simulink model "APF_CTL_VIS_Obs_2023a"  (R2023a)
settings: Solver=ode4  StartTime=0.0  StopTime=tsim  FixedStep=baseRate  RelTol=1e-6  AbsTol=1e-6
values from neighbouring files (symbols this model uses):
  A = [0 0 0 1 0 0 ... (first row only)    [CTL_NEW.m]    (also in UKF_SPOT.m = [1 0 0 dt 0 0)
  a = 25.028    [CTL_NEW.m]
  a1 = shape(1)    [Cardioid.m]    (also in Run_Initializer.m = 0.3)
  a2 = shape(2)    [Cardioid.m]    (also in Run_Initializer.m = 0.3)
  a3 = shape(3)    [Cardioid.m]    (also in Run_Initializer.m = 0.4)
  adadelta_epsilon = 1e-5    (= 1e-05)    [Run_Initializer.m]
  adadelta_gamma = 0.37    [Run_Initializer.m]
  adagrad_epsilon = 1e-8    (= 1e-08)    [Run_Initializer.m]
  adagrad_eta = 0.18    [Run_Initializer.m]
  adam_beta_1 = 0.99    [Run_Initializer.m]
  adam_beta_2 = 0.999    [Run_Initializer.m]
  adam_epsilon = 1e-2    (= 0.01)    [Run_Initializer.m]
  adam_eta = 0.0163    [Run_Initializer.m]
  adamax_beta_1 = 0.5    [Run_Initializer.m]
  adamax_beta_2 = 0.999    [Run_Initializer.m]
  adamax_eta = 0.014    [Run_Initializer.m]
  alpha_Black = 0.9    [UKF_SPOT.m]
  alpha_Blue = 0.9    [UKF_SPOT.m]
  Att_Mode = 0    [Run_Initializer.m]
  b1 = shape(4)    [Cardioid.m]    (also in Run_Initializer.m = 0.175)
  b2 = shape(5)    [Cardioid.m]    (also in Run_Initializer.m = 0.175)
  beta_Black = 2    [UKF_SPOT.m]
  beta_Blue = 20    [UKF_SPOT.m]
  Binv = inv(B)    [Run_Initializer.m]
  BLACK_end = [2, 1.4, deg2rad(368)]    [Run_Initializer.m]
  BLACK_ini = [2, 1.4, deg2rad(188), 0, 0, deg2rad(1.5)]    [Run_Initializer.m]
  BLUE_end = [1.3, 1.25, deg2rad(90)]    [Run_Initializer.m]
  BLUE_ini = [1.3, 1.25, deg2rad(270), 0, 0, deg2rad(-1.5)]    [Run_Initializer.m]
  drop_states_BLACK = BLACK_ini(1:3)    [Run_Initializer.m]
  drop_states_BLUE = BLUE_ini(1:3)    [Run_Initializer.m]
  drop_states_RED = RED_ini(1:3)    [Run_Initializer.m]
  dt = 0.01    [UKF_SPOT.m]
  end_time_black = 300    [Run_Initializer.m]
  end_time_blue = 300    [Run_Initializer.m]
  F_max = 0.22    [CTL_NEW.m]
  Gamma1_el = 0.12    [Run_Initializer.m]
  Gamma1_sh = 0.005    [Run_Initializer.m]
  Gamma1_wr = 0.025    [Run_Initializer.m]
  Gamma2_el = 5    [Run_Initializer.m]
  Gamma2_sh = 5    [Run_Initializer.m]
  Gamma2_wr = 5    [Run_Initializer.m]
  Gamma3_el = 10    [Run_Initializer.m]
  Gamma3_sh = 40    [Run_Initializer.m]
  Gamma3_wr = 40    [Run_Initializer.m]
  Gamma4_el = 0.039    [Run_Initializer.m]
  Gamma4_sh = 0.015    [Run_Initializer.m]
  Gamma4_wr = 0.029    [Run_Initializer.m]
  Gamma5_el = 800    [Run_Initializer.m]
  Gamma5_sh = 800    [Run_Initializer.m]
  Gamma5_wr = 800    [Run_Initializer.m]
  Gamma6_el = 0.000001    (= 1e-06)    [Run_Initializer.m]
  Gamma6_sh = 0.005    [Run_Initializer.m]
  Gamma6_wr = 0.02    [Run_Initializer.m]
  H = [1 0 0 0 0 0 ... (first row only)    [UKF_SPOT.m]
  home_states_BLACK = BLACK_ini(1:3)    [Run_Initializer.m]
  home_states_BLUE = BLUE_ini(1:3)    [Run_Initializer.m]
  home_states_RED = RED_ini(1:3)    [Run_Initializer.m]
  Hz = 0.01    [CTL_NEW.m]
  init_states_BLACK = BLACK_ini(1:3)    [Run_Initializer.m]
  init_states_BLUE = BLUE_ini(1:3)    [Run_Initializer.m]
  init_states_RED = RED_ini(1:3)    [Run_Initializer.m]
  J = IRED    [CTL_NEW.m]    (also in UKF_SPOT.m = 0.20184)
  k = lqr(A,B1,Q,R)    [CTL_NEW.m]
  k_1_0 = k(1,1)    [CTL_NEW.m]
  k_1_t_0 = k(3,3)    [CTL_NEW.m]
  k_2_0 = k(1,4)    [CTL_NEW.m]
  k_2_t_0 = k(3,6)    [CTL_NEW.m]
  K_a = diag([2 2 3.5])    [Run_Initializer.m]
  ka = 1    [Run_Initializer.m]
  Kd_elarm = 0.8    [Run_Initializer.m]
  Kd_sharm = 1.0    (= 1)    [Run_Initializer.m]
  Kd_t = 9.5    [CTL_NEW.m]    (also in Run_Initializer.m)
  Kd_wrarm = 0.6    [Run_Initializer.m]
  Kd_x = 28    [CTL_NEW.m]    (also in Run_Initializer.m)
  Kd_y = Kd_x    (= 28)    [CTL_NEW.m]    (also in Run_Initializer.m)
  Kp_elarm = 1.2    [Run_Initializer.m]
  Kp_sharm = 1.5    [Run_Initializer.m]
  Kp_t = 1    [CTL_NEW.m]    (also in Run_Initializer.m)
  Kp_wrarm = 2    [Run_Initializer.m]
  Kp_x = 3.5    [CTL_NEW.m]    (also in Run_Initializer.m)
  Kp_y = Kp_x    (= 3.5)    [CTL_NEW.m]    (also in Run_Initializer.m)
  kr = 2    [Run_Initializer.m]
  lambda1 = 0.4    [CTL_NEW.m]
  lambda12 = 0.4    [CTL_NEW.m]
  lambda12_t = 0.05    [CTL_NEW.m]
  lambda1_t = 0.05    [CTL_NEW.m]
  lambda2 = 0.4    [CTL_NEW.m]
  lambda2_t = 0.05    [CTL_NEW.m]
  lamda_Black = (alpha_Black^2)*(N + kappa_Black) - N    (= 15.06)    [UKF_SPOT.m]
  lamda_Blue = (alpha_Blue^2)*(N + kappa_Blue) - N    (= 6.96)    [UKF_SPOT.m]
  m = mRED    [CTL_NEW.m]    (also in UKF_SPOT.m = 11.21)
  method = 1    [UKF_SPOT.m]
  Method = 8    [Run_Initializer.m]
  momentum_eta = 0.7    [Run_Initializer.m]
  momentum_gamma = 0.7    [Run_Initializer.m]
  nesterov_eta = 0.6    [Run_Initializer.m]
  nesterov_gamma = 0.3    [Run_Initializer.m]
  Nmat = diag([1 1 1])    [Run_Initializer.m]
  p = 0.4    [CTL_NEW.m]
  P_b = diag([45 45 0])    [Run_Initializer.m]
  P_IC_Black = 0.2*eye(6)    [UKF_SPOT.m]
  P_IC_Blue = 0.2*eye(6)    [UKF_SPOT.m]
  p_t = 0.05    [CTL_NEW.m]
  psi = 1    [Run_Initializer.m]
  PWMFreq = 5    [Run_Initializer.m]
  Q = [w 0 0 0 0 0 ... (first row only)    [CTL_NEW.m]
  Q_a = diag([5, 5, 0])    [Run_Initializer.m]
  Q_b = diag([0.0125, 0.0125, 0.05])    [Run_Initializer.m]
  Q_Black = [0.0000005 0 0 0 0 0 ... (first row only)    [UKF_SPOT.m]
  Q_Blue = [0.000075 0 0 0 0 0 ... (first row only)    [UKF_SPOT.m]
  R = [r 0 0 ... (first row only)    [CTL_NEW.m]
  R_Black = [variance 0 0 ... (first row only)    [UKF_SPOT.m]
  R_Blue = [variance 0 0 ... (first row only)    [UKF_SPOT.m]
  r_hold = 0.427    [Run_Initializer.m]
  r_off = 0.165    [Run_Initializer.m]
  RED_ini = [2.7, 0.4, deg2rad(135+360), 0, 0, 0]    [Run_Initializer.m]
  Red_Rate = 0.025    [CTL_NEW.m]
  RMSprop_epsilon = 1e-8    (= 1e-08)    [Run_Initializer.m]
  RMSprop_eta = 0.025    [Run_Initializer.m]
  RMSprop_gamma = 0.9    [Run_Initializer.m]
  ... (+11 more)
undefined symbols (not defined in the file or in its folder): alpha, alpha_m, alphap, alphat, Am, b, b0, b3, baseRate, beta, Bm, c, Cm, d, DiscIntNeverNeededParam, Dm, drop_states_ARM, epsilon, F_Black_X_nominal, F_Black_Y_nominal, F_Blue_X_nominal, F_Blue_Y_nominal, F_red_X_nominal, F_red_Y_nominal, F_thrusters_BLACK, F_thrusters_BLUE, F_thrusters_RED, IBLACK, IBLUE, IDIST, IEE, IPROX, IRED, K, k1, k1t, k2, k2t, K_t, Kd_tb, Kd_tblue, Kd_tr, Kd_xb, Kd_xblue, Kd_xr, Kd_yb, Kd_yblue, Kd_yr, Kp_tb, Kp_tblue, Kp_tr, Kp_xb, Kp_xblue, Kp_xr, Kp_yb, Kp_yblue, Kp_yr, lamda ... (+34)
libraries: nvidiaSharedBlocks x10, MainLibrary x4, dspsigops x4, simulink x2, etargetslib x1
(part 4 of 15)

== system APF_CTL_VIS_Obs_2023a/Phase #2: Initial Position/Change BLACK Behavior/Custom Discrete PD (X-Position) ==
  ex : Inport
  Sum3 : Sum
  kd_xb : Gain  Gain=Kd_xb
  kp_xb : Gain  Gain=Kp_xb
  "x_dot -> x1" : Subsystem
  Fx : Outport  VectorParamsAs1DForOutWhenUnconnected=off
  wires:
  kd_xb/1 -> Sum3/1
  ex/1 -> "x_dot -> x1"/1(y(t)), kp_xb/1
  kp_xb/1 -> Sum3/2
  "x_dot -> x1"/1(dy(t)/dt) -> kd_xb/1
  Sum3/1 -> Fx/1

== system APF_CTL_VIS_Obs_2023a/Phase #2: Initial Position/Change BLACK Behavior/Custom Discrete PD (Y-Position) ==
  ey : Inport
  Sum3 : Sum
  kd_yb : Gain  Gain=Kd_yb
  kp_yb : Gain  Gain=Kp_yb
  "x_dot -> x1" : Subsystem
  Fy : Outport  VectorParamsAs1DForOutWhenUnconnected=off
  wires:
  kd_yb/1 -> Sum3/1
  Sum3/1 -> Fy/1
  kp_yb/1 -> Sum3/2
  "x_dot -> x1"/1(dy(t)/dt) -> kd_yb/1
  ey/1 -> "x_dot -> x1"/1(y(t)), kp_yb/1

== system APF_CTL_VIS_Obs_2023a/Phase #2: Initial Position/Change BLACK Behavior/Hough Control ==
  Ref : Inport
  Act : Inport  Port=2
  MATLAB Function2 : MATLAB Function  TreatAsAtomicUnit=on
  MATLAB Function3 : MATLAB Function  TreatAsAtomicUnit=on
  MATLAB Function4 : MATLAB Function  TreatAsAtomicUnit=on
  Subtract2 : Sum  Inputs=+-
  Err : Outport  VectorParamsAs1DForOutWhenUnconnected=off
  wires:
  MATLAB Function4/1(e_out) -> Err/1
  MATLAB Function2/1(Oy) -> MATLAB Function4/1(Oy)
  Subtract2/1 -> MATLAB Function4/2(e_in)
  MATLAB Function2/2(Ox) -> Subtract2/1
  Act/1 -> MATLAB Function3/1(z)
  Ref/1 -> MATLAB Function2/1(z)
  MATLAB Function3/1(Ox) -> Subtract2/2

== system APF_CTL_VIS_Obs_2023a/Phase #2: Initial Position/Change BLUE Behavior/Custom Discrete PD (Attitude) ==
  ez : Inport
  Sum3 : Sum
  kd_tb : Gain  Gain=Kd_tblue
  kp_tb : Gain  Gain=Kp_tblue
  "x_dot -> x1" : Subsystem
  Tz : Outport  VectorParamsAs1DForOutWhenUnconnected=off
  wires:
  kd_tb/1 -> Sum3/1
  Sum3/1 -> Tz/1
  kp_tb/1 -> Sum3/2
  "x_dot -> x1"/1(dy(t)/dt) -> kd_tb/1
  ez/1 -> "x_dot -> x1"/1(y(t)), kp_tb/1

== system APF_CTL_VIS_Obs_2023a/Phase #2: Initial Position/Change BLUE Behavior/Custom Discrete PD (X-Position) ==
  ex : Inport
  Sum3 : Sum
  kd_xb : Gain  Gain=Kd_xblue
  kp_xb : Gain  Gain=Kp_xblue
  "x_dot -> x1" : Subsystem
  Fx : Outport  VectorParamsAs1DForOutWhenUnconnected=off
  wires:
  kd_xb/1 -> Sum3/1
  ex/1 -> "x_dot -> x1"/1(y(t)), kp_xb/1
  kp_xb/1 -> Sum3/2
  "x_dot -> x1"/1(dy(t)/dt) -> kd_xb/1
  Sum3/1 -> Fx/1

== system APF_CTL_VIS_Obs_2023a/Phase #2: Initial Position/Change BLUE Behavior/Custom Discrete PD (Y-Position) ==
  ey : Inport
  Sum3 : Sum
  kd_yb : Gain  Gain=Kd_yblue
  kp_yb : Gain  Gain=Kp_yblue
  "x_dot -> x1" : Subsystem
  Fy : Outport  VectorParamsAs1DForOutWhenUnconnected=off
  wires:
  kd_yb/1 -> Sum3/1
  Sum3/1 -> Fy/1
  kp_yb/1 -> Sum3/2
  "x_dot -> x1"/1(dy(t)/dt) -> kd_yb/1
  ey/1 -> "x_dot -> x1"/1(y(t)), kp_yb/1

== system APF_CTL_VIS_Obs_2023a/Phase #2: Initial Position/Change BLUE Behavior/Hough Control ==
  Ref : Inport
  Act : Inport  Port=2
  MATLAB Function2 : MATLAB Function  TreatAsAtomicUnit=on
  MATLAB Function3 : MATLAB Function  TreatAsAtomicUnit=on
  MATLAB Function4 : MATLAB Function  TreatAsAtomicUnit=on
  Subtract2 : Sum  Inputs=+-
  Err : Outport  VectorParamsAs1DForOutWhenUnconnected=off
  wires:
  MATLAB Function4/1(e_out) -> Err/1
  MATLAB Function2/1(Oy) -> MATLAB Function4/1(Oy)
  Subtract2/1 -> MATLAB Function4/2(e_in)
  MATLAB Function2/2(Ox) -> Subtract2/1
  Act/1 -> MATLAB Function3/1(z)
  Ref/1 -> MATLAB Function2/1(z)
  MATLAB Function3/1(Ox) -> Subtract2/2

== system APF_CTL_VIS_Obs_2023a/Phase #2: Initial Position/Change RED Behavior/Custom Discrete PD (Attitude) ==
  ez : Inport
  Sum3 : Sum
  kd_tr : Gain  Gain=Kd_tr
  kp_tr : Gain  Gain=Kp_tr
  "x_dot -> x2" : Subsystem
  Tz : Outport  VectorParamsAs1DForOutWhenUnconnected=off
  wires:
  kd_tr/1 -> Sum3/1
  Sum3/1 -> Tz/1
  kp_tr/1 -> Sum3/2
  "x_dot -> x2"/1(dy(t)/dt) -> kd_tr/1
  ez/1 -> "x_dot -> x2"/1(y(t)), kp_tr/1

== system APF_CTL_VIS_Obs_2023a/Phase #2: Initial Position/Change RED Behavior/Custom Discrete PD (X-Position) ==
  ex : Inport
  Sum3 : Sum
  kd_xr : Gain  Gain=Kd_xr
  kp_xr : Gain  Gain=Kp_xr
  "x_dot -> x2" : Subsystem
  Fx : Outport  VectorParamsAs1DForOutWhenUnconnected=off
  wires:
  kd_xr/1 -> Sum3/1
  ex/1 -> "x_dot -> x2"/1(y(t)), kp_xr/1
  kp_xr/1 -> Sum3/2
  "x_dot -> x2"/1(dy(t)/dt) -> kd_xr/1
  Sum3/1 -> Fx/1

== system APF_CTL_VIS_Obs_2023a/Phase #2: Initial Position/Change RED Behavior/Custom Discrete PD (Y-Position) ==
  ey : Inport
  Sum3 : Sum
  kd_yr : Gain  Gain=Kd_yr
  kp_yr : Gain  Gain=Kp_yr
  "x_dot -> x2" : Subsystem
  Fy : Outport  VectorParamsAs1DForOutWhenUnconnected=off
  wires:
  kd_yr/1 -> Sum3/1
  Sum3/1 -> Fy/1
  kp_yr/1 -> Sum3/2
  "x_dot -> x2"/1(dy(t)/dt) -> kd_yr/1
  ey/1 -> "x_dot -> x2"/1(y(t)), kp_yr/1

== system APF_CTL_VIS_Obs_2023a/Phase #2: Initial Position/Change RED Behavior/Hough Control ==
  Ref : Inport
  Act : Inport  Port=2
  MATLAB Function2 : MATLAB Function  TreatAsAtomicUnit=on
  MATLAB Function3 : MATLAB Function  TreatAsAtomicUnit=on
  MATLAB Function4 : MATLAB Function  TreatAsAtomicUnit=on
  Subtract2 : Sum  Inputs=+-
  Err : Outport  VectorParamsAs1DForOutWhenUnconnected=off
  wires:
  MATLAB Function4/1(e_out) -> Err/1
  MATLAB Function2/1(Oy) -> MATLAB Function4/1(Oy)
  Subtract2/1 -> MATLAB Function4/2(e_in)
  MATLAB Function2/2(Ox) -> Subtract2/1
  Act/1 -> MATLAB Function3/1(z)
  Ref/1 -> MATLAB Function2/1(z)
  MATLAB Function3/1(Ox) -> Subtract2/2

== system APF_CTL_VIS_Obs_2023a/Phase #2: Initial Position/Change RED Behavior/RED+ARM ==
  note: ARM Control Law - RED
  note: This section is reserved for any control law for the robotic manipulator.
  Action Port : ActionPort  ActionPortLabel=if(u1 == 4 | u1 == 5 | u1 == 10 | u1 == 11)
  Constant4 : Constant  Value=pi/2
  Constant5 : Constant  Value=pi/2
  Constant6 : Constant  Value=0
  Constant7 : Constant
  Data Store Read1 : DataStoreRead  DataStoreName=isSim  IndexOptions=Index vector (dialog)  Indices=1  OutputSizes=1
  Data Store Write : DataStoreWrite  DataStoreName=RED_Shoulder_Command  IndexOptions=Index vector (dialog)  Indices=1  OutputSizes=1
  Data Store Write1 : DataStoreWrite  DataStoreName=RED_Elbow_Command  IndexOptions=Index vector (dialog)  Indices=1  OutputSizes=1
  Data Store Write2 : DataStoreWrite  DataStoreName=RED_Wrist_Command  IndexOptions=Index vector (dialog)  Indices=1  OutputSizes=1
  Data Store Write3 : DataStoreWrite  DataStoreName=RED_ARM_Control_Mode  IndexOptions=Index vector (dialog)  Indices=1  OutputSizes=1
  "If 'simMode' set to '1', then this is a simulation and the dynamics will be simulated. Otherwise, this is an experiment, and the simulation will not be run." : If  IfExpression=u1 == 1
  Merge : Merge
  Merge1 : Merge
  Merge2 : Merge
  Passthrough for Experiment : Subsystem  TreatAsAtomicUnit=on
  Simulated Position Controller : Subsystem  TreatAsAtomicUnit=on
  wires:
  Constant7/1 -> Data Store Write3/1
  Constant6/1 -> Passthrough for Experiment/3(q3_desired), Simulated Position Controller/3(q3_desired)
  Constant4/1 -> Passthrough for Experiment/1(q1_desired), Simulated Position Controller/1(q1_desired)
  Constant5/1 -> Passthrough for Experiment/2(q2_desired), Simulated Position Controller/2(q2_desired)
  Data Store Read1/1 -> "If 'simMode' set to '1', then this is a simulation and the dynamics will be simulated. Otherwise, this is an experiment, and the simulation will not be run."/1
  "If 'simMode' set to '1', then this is a simulation and the dynamics will be simulated. Otherwise, this is an experiment, and the simulation will not be run."/1 -> Simulated Position Controller/Action
  "If 'simMode' set to '1', then this is a simulation and the dynamics will be simulated. Otherwise, this is an experiment, and the simulation will not be run."/2 -> Passthrough for Experiment/Action
  Simulated Position Controller/1(q1_command) -> Merge/1
  Passthrough for Experiment/1(q1_command) -> Merge/2
  Merge/1 -> Data Store Write/1
  Simulated Position Controller/2(q2_command) -> Merge1/1
  Merge1/1 -> Data Store Write1/1
  Passthrough for Experiment/2(q2_command) -> Merge1/2
  Simulated Position Controller/3(q3_command) -> Merge2/1
  Passthrough for Experiment/3(q3_command) -> Merge2/2
  Merge2/1 -> Data Store Write2/1

== system APF_CTL_VIS_Obs_2023a/Phase #3: Experiment/Change BLACK Behavior/Sub-Phase #1 ==
  note: PD Control Law - BLACK
  note: Additional Blocks
  note: A simple PD control law is used here to command the platform to it's initial position, as defined in the initializer.
  note: Additional blocks are stored here.
  Action Port : ActionPort  ActionPortLabel=if(u1 < u2)
  BLACK_Fx : DataStoreWrite  DataStoreName=BLACK_Fx  IndexOptions=Index vector (dialog)  Indices=1  OutputSizes=1
  BLACK_Fy : DataStoreWrite  DataStoreName=BLACK_Fy  IndexOptions=Index vector (dialog)  Indices=1  OutputSizes=1
  BLACK_Px : DataStoreRead  DataStoreName=BLACK_Px  IndexOptions=Index vector (dialog)  Indices=1  OutputSizes=1
  "BLACK_Py " : DataStoreRead  DataStoreName=BLACK_Py  IndexOptions=Index vector (dialog)  Indices=1  OutputSizes=1
  BLACK_Rz : DataStoreRead  DataStoreName=BLACK_Rz  IndexOptions=Index vector (dialog)  Indices=1  OutputSizes=1
  BLACK_Rz Desired : Subsystem
  BLACK_Tz : DataStoreWrite  DataStoreName=BLACK_Tz  IndexOptions=Index vector (dialog)  Indices=1  OutputSizes=1
  Custom Discrete PD (Attitude) : Subsystem
  Custom Discrete PD (X-Position) : Subsystem
  Custom Discrete PD (Y-Position) : Subsystem
  Data Store Write3 : DataStoreWrite  DataStoreName=Float_State  IndexOptions=Index vector (dialog)  Indices=1  OutputSizes=1
  Desired X-Position (BLACK) : Constant  Value=xLength/2  SampleTime=-1
  Desired Y-Position (BLACK) : Constant  Value=yLength/2  SampleTime=-1
  Hough Control : Subsystem
  Puck State : Constant
  Subtract : Sum  Inputs=+-
  Subtract1 : Sum  Inputs=+-
  wires:
  Puck State/1 -> Data Store Write3/1
  "BLACK_Py "/1 -> Subtract1/2
  Desired X-Position (BLACK)/1 -> Subtract/1
  BLACK_Rz Desired/1(Out1) -> Hough Control/1(Ref)
  Custom Discrete PD (X-Position)/1(Fx) -> BLACK_Fx/1
  Desired Y-Position (BLACK)/1 -> Subtract1/1
  Hough Control/1(Err) -> Custom Discrete PD (Attitude)/1(ez)
  Subtract/1 -> Custom Discrete PD (X-Position)/1(ex)
  Custom Discrete PD (Y-Position)/1(Fy) -> BLACK_Fy/1
  Subtract1/1 -> Custom Discrete PD (Y-Position)/1(ey)
  Custom Discrete PD (Attitude)/1(Tz) -> BLACK_Tz/1
  BLACK_Rz/1 -> Hough Control/2(Act)
  BLACK_Px/1 -> Subtract/2

== system APF_CTL_VIS_Obs_2023a/Phase #3: Experiment/Change BLACK Behavior/Sub-Phase #2  ==
  note: PD Control Law - BLACK
  note: Additional Blocks
  note: Additional blocks are stored here.
  Action Port : ActionPort  ActionPortLabel=elseif((u1 < u3 & u1 >= u2))
  BLACK_Fx : DataStoreWrite  DataStoreName=BLACK_Fx  IndexOptions=Index vector (dialog)  Indices=1  OutputSizes=1
  BLACK_Fy : DataStoreWrite  DataStoreName=BLACK_Fy  IndexOptions=Index vector (dialog)  Indices=1  OutputSizes=1
  BLACK_Px : DataStoreRead  DataStoreName=BLACK_Px  IndexOptions=Index vector (dialog)  Indices=1  OutputSizes=1
  "BLACK_Py " : DataStoreRead  DataStoreName=BLACK_Py  IndexOptions=Index vector (dialog)  Indices=1  OutputSizes=1
  BLACK_Rz : DataStoreRead  DataStoreName=BLACK_Rz  IndexOptions=Index vector (dialog)  Indices=1  OutputSizes=1
  BLACK_Rz Desired : Subsystem
  BLACK_Tz : DataStoreWrite  DataStoreName=BLACK_Tz  IndexOptions=Index vector (dialog)  Indices=1  OutputSizes=1
  Custom Discrete PD (Attitude) : Subsystem
  Custom Discrete PD (X-Position) : Subsystem
  Custom Discrete PD (Y-Position) : Subsystem
  Data Store Write3 : DataStoreWrite  DataStoreName=Float_State  IndexOptions=Index vector (dialog)  Indices=1  OutputSizes=1
  Desired X-Position (BLACK) : Constant  Value=xLength/2  SampleTime=-1
  Desired Y-Position (BLACK) : Constant  Value=yLength/2  SampleTime=-1
  Hough Control : Subsystem
  Puck State : Constant
  Subtract : Sum  Inputs=+-
  Subtract1 : Sum  Inputs=+-
  wires:
  Puck State/1 -> Data Store Write3/1
  BLACK_Px/1 -> Subtract/2
  Custom Discrete PD (Y-Position)/1(Fy) -> BLACK_Fy/1
  Subtract/1 -> Custom Discrete PD (X-Position)/1(ex)
  Desired Y-Position (BLACK)/1 -> Subtract1/1
  Custom Discrete PD (Attitude)/1(Tz) -> BLACK_Tz/1
  Subtract1/1 -> Custom Discrete PD (Y-Position)/1(ey)
  BLACK_Rz/1 -> Hough Control/2(Act)
  Custom Discrete PD (X-Position)/1(Fx) -> BLACK_Fx/1
  Hough Control/1(Err) -> Custom Discrete PD (Attitude)/1(ez)
  "BLACK_Py "/1 -> Subtract1/2
  Desired X-Position (BLACK)/1 -> Subtract/1
  BLACK_Rz Desired/1(Out1) -> Hough Control/1(Ref)

== system APF_CTL_VIS_Obs_2023a/Phase #3: Experiment/Change BLACK Behavior/Sub-Phase #3  ==
  note: PD Control Law - BLACK
  note: Additional Blocks
  note: Additional blocks are stored here.
  Action Port : ActionPort  ActionPortLabel=elseif((u1 < u4 & u1 >= u3))
  BLACK_Fx : DataStoreWrite  DataStoreName=BLACK_Fx  IndexOptions=Index vector (dialog)  Indices=1  OutputSizes=1
  BLACK_Fy : DataStoreWrite  DataStoreName=BLACK_Fy  IndexOptions=Index vector (dialog)  Indices=1  OutputSizes=1
  BLACK_Px : DataStoreRead  DataStoreName=BLACK_Px  IndexOptions=Index vector (dialog)  Indices=1  OutputSizes=1
  "BLACK_Py " : DataStoreRead  DataStoreName=BLACK_Py  IndexOptions=Index vector (dialog)  Indices=1  OutputSizes=1
  BLACK_Rz : DataStoreRead  DataStoreName=BLACK_Rz  IndexOptions=Index vector (dialog)  Indices=1  OutputSizes=1
  BLACK_Rz Desired : Subsystem
  BLACK_Tz : DataStoreWrite  DataStoreName=BLACK_Tz  IndexOptions=Index vector (dialog)  Indices=1  OutputSizes=1
  Custom Discrete PD (Attitude) : Subsystem
  Custom Discrete PD (X-Position) : Subsystem
  Custom Discrete PD (Y-Position) : Subsystem
  Data Store Write3 : DataStoreWrite  DataStoreName=Float_State  IndexOptions=Index vector (dialog)  Indices=1  OutputSizes=1
  Desired X-Position (BLACK) : Constant  Value=xLength/2  SampleTime=-1
  Desired Y-Position (BLACK) : Constant  Value=yLength/2  SampleTime=-1
  Hough Control : Subsystem
  Puck State : Constant
  Subtract : Sum  Inputs=+-
  Subtract1 : Sum  Inputs=+-
  wires:
  Puck State/1 -> Data Store Write3/1
  BLACK_Px/1 -> Subtract/2
  Custom Discrete PD (Y-Position)/1(Fy) -> BLACK_Fy/1
  Subtract/1 -> Custom Discrete PD (X-Position)/1(ex)
  Desired Y-Position (BLACK)/1 -> Subtract1/1
  Custom Discrete PD (Attitude)/1(Tz) -> BLACK_Tz/1
  Subtract1/1 -> Custom Discrete PD (Y-Position)/1(ey)
  BLACK_Rz/1 -> Hough Control/2(Act)
  Custom Discrete PD (X-Position)/1(Fx) -> BLACK_Fx/1
  Hough Control/1(Err) -> Custom Discrete PD (Attitude)/1(ez)
  "BLACK_Py "/1 -> Subtract1/2
  Desired X-Position (BLACK)/1 -> Subtract/1
  BLACK_Rz Desired/1(Out1) -> Hough Control/1(Ref)

== system APF_CTL_VIS_Obs_2023a/Phase #3: Experiment/Change BLACK Behavior/Sub-Phase #4 ==
  note: PD Control Law - BLACK
  note: Additional Blocks
  note: A simple PD control law is used here to command the platform to it's initial position, as defined in the initializer.
  note: Additional blocks are stored here.
  Action Port : ActionPort  ActionPortLabel=elseif( (u1 < u5 & u1 >= u4))
  BLACK_Fx : DataStoreWrite  DataStoreName=BLACK_Fx  IndexOptions=Index vector (dialog)  Indices=1  OutputSizes=1
  BLACK_Fy : DataStoreWrite  DataStoreName=BLACK_Fy  IndexOptions=Index vector (dialog)  Indices=1  OutputSizes=1
  BLACK_Px : DataStoreRead  DataStoreName=BLACK_Px  IndexOptions=Index vector (dialog)  Indices=1  OutputSizes=1
  "BLACK_Py " : DataStoreRead  DataStoreName=BLACK_Py  IndexOptions=Index vector (dialog)  Indices=1  OutputSizes=1
  BLACK_Rz : DataStoreRead  DataStoreName=BLACK_Rz  IndexOptions=Index vector (dialog)  Indices=1  OutputSizes=1
  BLACK_RzD : Subsystem  Commented=on
  BLACK_Tz : DataStoreWrite  DataStoreName=BLACK_Tz  IndexOptions=Index vector (dialog)  Indices=1  OutputSizes=1
  Custom Discrete PD (Attitude) : Subsystem
  Custom Discrete PD (X-Position) : Subsystem
  Custom Discrete PD (Y-Position) : Subsystem
  Data Store Write3 : DataStoreWrite  DataStoreName=Float_State  IndexOptions=Index vector (dialog)  Indices=1  OutputSizes=1
  Hough Control : Subsystem
  Motion X1 : Subsystem
  Motion Y1 : Subsystem
  Motion Z1 : Subsystem
  Puck State : Constant
  Subtract : Sum  Inputs=+-
  Subtract1 : Sum  Inputs=+-
  wires:
  Puck State/1 -> Data Store Write3/1
  BLACK_Rz/1 -> Hough Control/2(Act)
  Subtract1/1 -> Custom Discrete PD (Y-Position)/1(ey)
  Hough Control/1(Err) -> Custom Discrete PD (Attitude)/1(ez)
  "BLACK_Py "/1 -> Subtract1/2
  BLACK_Px/1 -> Subtract/2
  Subtract/1 -> Custom Discrete PD (X-Position)/1(ex)
  Custom Discrete PD (Attitude)/1(Tz) -> BLACK_Tz/1
  Custom Discrete PD (Y-Position)/1(Fy) -> BLACK_Fy/1
  Custom Discrete PD (X-Position)/1(Fx) -> BLACK_Fx/1
  Motion X1/1(Out1) -> Subtract/1
  Motion Y1/1(Out1) -> Subtract1/1
  Motion Z1/1(Ref) -> Hough Control/1(Ref)

== system APF_CTL_VIS_Obs_2023a/Phase #3: Experiment/Change BLUE Behavior/Sub-Phase #1 ==
  note: PD Control Law - BLUE
  note: A simple PD control law is used here to command the platform to it's initial position, as defined in the initializer.
  note: Additional Blocks
  note: Additional blocks are stored here.
  Action Port : ActionPort  ActionPortLabel=if(u1 < u2)
  BLUE_Fx : DataStoreWrite  DataStoreName=BLUE_Fx  IndexOptions=Index vector (dialog)  Indices=1  OutputSizes=1
  BLUE_Fy : DataStoreWrite  DataStoreName=BLUE_Fy  IndexOptions=Index vector (dialog)  Indices=1  OutputSizes=1
  BLUE_Px : DataStoreRead  DataStoreName=BLUE_Px  IndexOptions=Index vector (dialog)  Indices=1  OutputSizes=1
  "BLUE_Py " : DataStoreRead  DataStoreName=BLUE_Py  IndexOptions=Index vector (dialog)  Indices=1  OutputSizes=1
  BLUE_Rz : DataStoreRead  DataStoreName=BLUE_Rz  IndexOptions=Index vector (dialog)  Indices=1  OutputSizes=1
  BLUE_Rz Desired : Subsystem
  BLUE_Tz : DataStoreWrite  DataStoreName=BLUE_Tz  IndexOptions=Index vector (dialog)  Indices=1  OutputSizes=1
  Custom Discrete PD (Attitude) : Subsystem
  Custom Discrete PD (X-Position) : Subsystem
  Custom Discrete PD (Y-Position) : Subsystem
  Data Store Write1 : DataStoreWrite  DataStoreName=Float_State  IndexOptions=Index vector (dialog)  Indices=1  OutputSizes=1
  Hough Control : Subsystem
  MATLAB Function2 : MATLAB Function  TreatAsAtomicUnit=on
  MATLAB Function3 : MATLAB Function  TreatAsAtomicUnit=on
  Puck State : Constant
  Subsystem2 : Subsystem
  Subtract : Sum  Inputs=+-
  Subtract1 : Sum  Inputs=+-
  wires:
  Puck State/1 -> Data Store Write1/1
  Custom Discrete PD (Attitude)/1(Tz) -> BLUE_Tz/1
  MATLAB Function3/1(y) -> Subtract1/1
  MATLAB Function2/1(x) -> Subtract/1
  Hough Control/1(Err) -> Custom Discrete PD (Attitude)/1(ez)
  BLUE_Rz/1 -> Hough Control/2(Act)
  Custom Discrete PD (Y-Position)/1(Fy) -> BLUE_Fy/1
  Subtract/1 -> Custom Discrete PD (X-Position)/1(ex)
  BLUE_Px/1 -> Subtract/2
  Custom Discrete PD (X-Position)/1(Fx) -> BLUE_Fx/1
  Subsystem2/1(Out1) -> MATLAB Function2/1(t), MATLAB Function3/1(t)
  Subtract1/1 -> Custom Discrete PD (Y-Position)/1(ey)
  "BLUE_Py "/1 -> Subtract1/2
  BLUE_Rz Desired/1(Ref) -> Hough Control/1(Ref)

== system APF_CTL_VIS_Obs_2023a/Phase #3: Experiment/Change BLUE Behavior/Sub-Phase #2  ==
  note: Additional blocks are stored here.
  note: A simple PD control law is used here to command the platform to it's initial position, as defined in the initializer.
  note: Additional Blocks
  note: PD Control Law - BLUE
  Action Port : ActionPort  ActionPortLabel=elseif((u1 < u3 & u1 >= u2))
  BLUE_Fx : DataStoreWrite  DataStoreName=BLUE_Fx  IndexOptions=Index vector (dialog)  Indices=1  OutputSizes=1
  BLUE_Fy : DataStoreWrite  DataStoreName=BLUE_Fy  IndexOptions=Index vector (dialog)  Indices=1  OutputSizes=1
  BLUE_Px : DataStoreRead  DataStoreName=BLUE_Px  IndexOptions=Index vector (dialog)  Indices=1  OutputSizes=1
  "BLUE_Py " : DataStoreRead  DataStoreName=BLUE_Py  IndexOptions=Index vector (dialog)  Indices=1  OutputSizes=1
  BLUE_Rz : DataStoreRead  DataStoreName=BLUE_Rz  IndexOptions=Index vector (dialog)  Indices=1  OutputSizes=1
  BLUE_Rz Desired : Subsystem
  BLUE_Tz : DataStoreWrite  DataStoreName=BLUE_Tz  IndexOptions=Index vector (dialog)  Indices=1  OutputSizes=1
  Custom Discrete PD (Attitude) : Subsystem
  Custom Discrete PD (X-Position) : Subsystem
  Custom Discrete PD (Y-Position) : Subsystem
  Data Store Write1 : DataStoreWrite  DataStoreName=Float_State  IndexOptions=Index vector (dialog)  Indices=1  OutputSizes=1
  Hough Control : Subsystem
  MATLAB Function2 : MATLAB Function  TreatAsAtomicUnit=on
  MATLAB Function3 : MATLAB Function  TreatAsAtomicUnit=on
  Puck State : Constant
  Subsystem2 : Subsystem
  Subtract : Sum  Inputs=+-
  Subtract1 : Sum  Inputs=+-
  wires:
  Puck State/1 -> Data Store Write1/1
  BLUE_Rz/1 -> Hough Control/2(Act)
  BLUE_Rz Desired/1(Ref) -> Hough Control/1(Ref)
  Custom Discrete PD (Y-Position)/1(Fy) -> BLUE_Fy/1
  Subtract/1 -> Custom Discrete PD (X-Position)/1(ex)
  Subtract1/1 -> Custom Discrete PD (Y-Position)/1(ey)
  BLUE_Px/1 -> Subtract/2
  Custom Discrete PD (X-Position)/1(Fx) -> BLUE_Fx/1
  "BLUE_Py "/1 -> Subtract1/2
  Subsystem2/1(Out1) -> MATLAB Function2/1(t), MATLAB Function3/1(t)
  MATLAB Function2/1(x) -> Subtract/1
  Hough Control/1(Err) -> Custom Discrete PD (Attitude)/1(ez)
  MATLAB Function3/1(y) -> Subtract1/1
  Custom Discrete PD (Attitude)/1(Tz) -> BLUE_Tz/1

== system APF_CTL_VIS_Obs_2023a/Phase #3: Experiment/Change BLUE Behavior/Sub-Phase #3  ==
  note: Additional blocks are stored here.
  note: A simple PD control law is used here to command the platform to it's initial position, as defined in the initializer.
  note: Additional Blocks
  note: PD Control Law - BLUE
  Action Port : ActionPort  ActionPortLabel=elseif((u1 < u4 & u1 >= u3))
  BLUE_Fx : DataStoreWrite  DataStoreName=BLUE_Fx  IndexOptions=Index vector (dialog)  Indices=1  OutputSizes=1
  BLUE_Fy : DataStoreWrite  DataStoreName=BLUE_Fy  IndexOptions=Index vector (dialog)  Indices=1  OutputSizes=1
  BLUE_Px : DataStoreRead  DataStoreName=BLUE_Px  IndexOptions=Index vector (dialog)  Indices=1  OutputSizes=1
  "BLUE_Py " : DataStoreRead  DataStoreName=BLUE_Py  IndexOptions=Index vector (dialog)  Indices=1  OutputSizes=1
  BLUE_Rz : DataStoreRead  DataStoreName=BLUE_Rz  IndexOptions=Index vector (dialog)  Indices=1  OutputSizes=1
  BLUE_Rz Desired : Subsystem
  BLUE_Tz : DataStoreWrite  DataStoreName=BLUE_Tz  IndexOptions=Index vector (dialog)  Indices=1  OutputSizes=1
  Custom Discrete PD (Attitude) : Subsystem
  Custom Discrete PD (X-Position) : Subsystem
  Custom Discrete PD (Y-Position) : Subsystem
  Data Store Write1 : DataStoreWrite  DataStoreName=Float_State  IndexOptions=Index vector (dialog)  Indices=1  OutputSizes=1
  Hough Control : Subsystem
  MATLAB Function2 : MATLAB Function  TreatAsAtomicUnit=on
  MATLAB Function3 : MATLAB Function  TreatAsAtomicUnit=on
  Puck State : Constant
  Subsystem2 : Subsystem
  Subtract : Sum  Inputs=+-
  Subtract1 : Sum  Inputs=+-
  wires:
  Puck State/1 -> Data Store Write1/1
  BLUE_Rz/1 -> Hough Control/2(Act)
  BLUE_Rz Desired/1(Ref) -> Hough Control/1(Ref)
  Custom Discrete PD (Y-Position)/1(Fy) -> BLUE_Fy/1
  Subtract/1 -> Custom Discrete PD (X-Position)/1(ex)
  Subtract1/1 -> Custom Discrete PD (Y-Position)/1(ey)
  BLUE_Px/1 -> Subtract/2
  Custom Discrete PD (X-Position)/1(Fx) -> BLUE_Fx/1
  "BLUE_Py "/1 -> Subtract1/2
  Subsystem2/1(Out1) -> MATLAB Function2/1(t), MATLAB Function3/1(t)
  MATLAB Function2/1(x) -> Subtract/1
  Hough Control/1(Err) -> Custom Discrete PD (Attitude)/1(ez)
  MATLAB Function3/1(y) -> Subtract1/1
  Custom Discrete PD (Attitude)/1(Tz) -> BLUE_Tz/1

== system APF_CTL_VIS_Obs_2023a/Phase #3: Experiment/Change BLUE Behavior/Sub-Phase #4 ==
  note: Additional blocks are stored here.
  note: A simple PD control law is used here to command the platform to it's initial position, as defined in the initializer.
  note: Additional Blocks
  note: PD Control Law - BLUE
  Action Port : ActionPort  ActionPortLabel=elseif( (u1 < u5 & u1 >= u4))
  BLUE_Fx : DataStoreWrite  DataStoreName=BLUE_Fx  IndexOptions=Index vector (dialog)  Indices=1  OutputSizes=1
  BLUE_Fy : DataStoreWrite  DataStoreName=BLUE_Fy  IndexOptions=Index vector (dialog)  Indices=1  OutputSizes=1
  BLUE_Px : DataStoreRead  DataStoreName=BLUE_Px  IndexOptions=Index vector (dialog)  Indices=1  OutputSizes=1
  "BLUE_Py " : DataStoreRead  DataStoreName=BLUE_Py  IndexOptions=Index vector (dialog)  Indices=1  OutputSizes=1
  BLUE_Rz : DataStoreRead  Commented=on  DataStoreName=BLUE_Rz  IndexOptions=Index vector (dialog)  Indices=1  OutputSizes=1
  BLUE_Rz Desired : Subsystem  Commented=on
  BLUE_Tz : DataStoreWrite  DataStoreName=BLUE_Tz  IndexOptions=Index vector (dialog)  Indices=1  OutputSizes=1
  Custom Discrete PD (Attitude) : Subsystem
  Custom Discrete PD (X-Position) : Subsystem
  Custom Discrete PD (Y-Position) : Subsystem
  Data Store Read : DataStoreRead  DataStoreName=BLUE_Rz  IndexOptions=Index vector (dialog)  Indices=1  OutputSizes=1
  Data Store Write1 : DataStoreWrite  DataStoreName=Float_State  IndexOptions=Index vector (dialog)  Indices=1  OutputSizes=1
  Hough Control : Subsystem
  Motion X : Subsystem
  Motion Y : Subsystem
  Motion Z : Subsystem
  Puck State : Constant
  Subtract : Sum  Inputs=+-
  Subtract1 : Sum  Inputs=+-
  wires:
  Puck State/1 -> Data Store Write1/1
  Data Store Read/1 -> Hough Control/2(Act)
  Custom Discrete PD (Attitude)/1(Tz) -> BLUE_Tz/1
  Subtract1/1 -> Custom Discrete PD (Y-Position)/1(ey)
  Hough Control/1(Err) -> Custom Discrete PD (Attitude)/1(ez)
  Custom Discrete PD (X-Position)/1(Fx) -> BLUE_Fx/1
  BLUE_Px/1 -> Subtract/2
  Subtract/1 -> Custom Discrete PD (X-Position)/1(ex)
  Custom Discrete PD (Y-Position)/1(Fy) -> BLUE_Fy/1
  "BLUE_Py "/1 -> Subtract1/2
  Motion X/1(Out1) -> Subtract/1
  Motion Y/1(Out1) -> Subtract1/1
  Motion Z/1(Ref) -> Hough Control/1(Ref)

== system APF_CTL_VIS_Obs_2023a/Phase #3: Experiment/Change RED Behavior/Sub-Phase #1 ==
  note: PD Control Law - RED
  note: Additional Blocks
  note: Additional blocks are stored above. Note that to control attitude using the RW, simply replace RED_Tz with RED_Tz_RW.
  note: A simple PD control law is used here to command the platform to it's initial position, as defined in the initializer.
  note: ARM Control Law - RED
  Action Port : ActionPort  ActionPortLabel=if(u1 < u2)
  Constant1 : Constant  Value=0
  Constant4 : Constant  Value=platformSelection
  Custom Discrete PD (Attitude) : Subsystem
  Custom Discrete PD (X-Position) : Subsystem
  Custom Discrete PD (Y-Position) : Subsystem
  Data Store Write3 : DataStoreWrite  DataStoreName=Float_State  IndexOptions=Index vector (dialog)  Indices=1  OutputSizes=1
  Hough Control : Subsystem
  If : If  IfExpression=u1 == 4 | u1 == 5 | u1 == 10 | u1 == 11  ShowElse=off
  MATLAB Function : MATLAB Function  TreatAsAtomicUnit=on
  MATLAB Function1 : MATLAB Function  TreatAsAtomicUnit=on
  Puck State : Constant
  RED+ARM : Subsystem  TreatAsAtomicUnit=on
  RED_Fx : DataStoreWrite  DataStoreName=RED_Fx  IndexOptions=Index vector (dialog)  Indices=1  OutputSizes=1
  RED_Fy : DataStoreWrite  DataStoreName=RED_Fy  IndexOptions=Index vector (dialog)  Indices=1  OutputSizes=1
  RED_Px1 : DataStoreRead  DataStoreName=RED_Px  IndexOptions=Index vector (dialog)  Indices=1  OutputSizes=1
  "RED_Py " : DataStoreRead  DataStoreName=RED_Py  IndexOptions=Index vector (dialog)  Indices=1  OutputSizes=1
  RED_Rz : DataStoreRead  DataStoreName=RED_Rz  IndexOptions=Index vector (dialog)  Indices=1  OutputSizes=1
  RED_Rz Desired : Subsystem
  RED_Tz : DataStoreWrite  DataStoreName=RED_Tz  IndexOptions=Index vector (dialog)  Indices=1  OutputSizes=1
  RED_Tz_RW : DataStoreWrite  DataStoreName=RED_Tz_RW  IndexOptions=Index vector (dialog)  Indices=1  OutputSizes=1
  Subsystem1 : Subsystem
  Subtract : Sum  Inputs=+-
  Subtract2 : Sum  Inputs=+-
  wires:
  Constant1/1 -> RED_Tz_RW/1
  Puck State/1 -> Data Store Write3/1
  If/1 -> RED+ARM/Action
  Constant4/1 -> If/1
  Subsystem1/1(Out1) -> MATLAB Function/1(t), MATLAB Function1/1(t)
  Hough Control/1(Err) -> Custom Discrete PD (Attitude)/1(ez)
  "RED_Py "/1 -> Subtract2/2
  Custom Discrete PD (Y-Position)/1(Fy) -> RED_Fy/1
  Custom Discrete PD (Attitude)/1(Tz) -> RED_Tz/1
  RED_Px1/1 -> Subtract/2
  MATLAB Function/1(x) -> Subtract/1
  RED_Rz Desired/1(Ref) -> Hough Control/1(Ref)
  Custom Discrete PD (X-Position)/1(Fx) -> RED_Fx/1
  Subtract/1 -> Custom Discrete PD (X-Position)/1(ex)
  MATLAB Function1/1(y) -> Subtract2/1
  Subtract2/1 -> Custom Discrete PD (Y-Position)/1(ey)
  RED_Rz/1 -> Hough Control/2(Act)

== system APF_CTL_VIS_Obs_2023a/Phase #3: Experiment/Change RED Behavior/Sub-Phase #2  ==
  note: PD Control Law - RED
  note: Additional Blocks
  note: Additional blocks are stored above. Note that to control attitude using the RW, simply replace RED_Tz with RED_Tz_RW.
  note: ARM Control Law - RED
  Action Port : ActionPort  ActionPortLabel=elseif((u1 < u3 & u1 >= u2))
  Constant1 : Constant  Value=0
  Constant4 : Constant  Value=platformSelection
  Custom Discrete PD (Attitude) : Subsystem
  Custom Discrete PD (X-Position) : Subsystem
  Custom Discrete PD (Y-Position) : Subsystem
  Data Store Write3 : DataStoreWrite  DataStoreName=Float_State  IndexOptions=Index vector (dialog)  Indices=1  OutputSizes=1
  Hough Control : Subsystem
  If : If  IfExpression=u1 == 4 | u1 == 5 | u1 == 10 | u1 == 11  ShowElse=off
  MATLAB Function : MATLAB Function  TreatAsAtomicUnit=on
  MATLAB Function1 : MATLAB Function  TreatAsAtomicUnit=on
  Puck State : Constant
  RED+ARM : Subsystem  TreatAsAtomicUnit=on
  RED_Fx : DataStoreWrite  DataStoreName=RED_Fx  IndexOptions=Index vector (dialog)  Indices=1  OutputSizes=1
  RED_Fy : DataStoreWrite  DataStoreName=RED_Fy  IndexOptions=Index vector (dialog)  Indices=1  OutputSizes=1
  RED_Px1 : DataStoreRead  DataStoreName=RED_Px  IndexOptions=Index vector (dialog)  Indices=1  OutputSizes=1
  "RED_Py " : DataStoreRead  DataStoreName=RED_Py  IndexOptions=Index vector (dialog)  Indices=1  OutputSizes=1
  RED_Rz : DataStoreRead  DataStoreName=RED_Rz  IndexOptions=Index vector (dialog)  Indices=1  OutputSizes=1
  RED_Rz Desired : Subsystem
  RED_Tz : DataStoreWrite  DataStoreName=RED_Tz  IndexOptions=Index vector (dialog)  Indices=1  OutputSizes=1
  RED_Tz_RW : DataStoreWrite  DataStoreName=RED_Tz_RW  IndexOptions=Index vector (dialog)  Indices=1  OutputSizes=1
  Subsystem1 : Subsystem
  Subtract : Sum  Inputs=+-
  Subtract2 : Sum  Inputs=+-
  wires:
  Constant1/1 -> RED_Tz_RW/1
  Puck State/1 -> Data Store Write3/1
  Subtract2/1 -> Custom Discrete PD (Y-Position)/1(ey)
  "RED_Py "/1 -> Subtract2/2
  RED_Rz Desired/1(Ref) -> Hough Control/1(Ref)
  MATLAB Function/1(x) -> Subtract/1
  RED_Rz/1 -> Hough Control/2(Act)
  Subtract/1 -> Custom Discrete PD (X-Position)/1(ex)
  MATLAB Function1/1(y) -> Subtract2/1
  Custom Discrete PD (Attitude)/1(Tz) -> RED_Tz/1
  RED_Px1/1 -> Subtract/2
  Subsystem1/1(Out1) -> MATLAB Function/1(t), MATLAB Function1/1(t)
  Custom Discrete PD (X-Position)/1(Fx) -> RED_Fx/1
  Hough Control/1(Err) -> Custom Discrete PD (Attitude)/1(ez)
  Custom Discrete PD (Y-Position)/1(Fy) -> RED_Fy/1
  If/1 -> RED+ARM/Action
  Constant4/1 -> If/1

== system APF_CTL_VIS_Obs_2023a/Phase #3: Experiment/Change RED Behavior/Sub-Phase #3  ==
  note: PD Control Law - RED
  note: Additional Blocks
  note: Additional blocks are stored above. Note that to control attitude using the RW, simply replace RED_Tz with RED_Tz_RW.
  note: ARM Control Law - RED
  Action Port : ActionPort  ActionPortLabel=elseif((u1 < u4 & u1 >= u3))
  Constant1 : Constant  Value=platformSelection
  Constant4 : Constant  Value=0
  Custom Discrete PD (Attitude) : Subsystem
  Custom Discrete PD (X-Position) : Subsystem
  Custom Discrete PD (Y-Position) : Subsystem
  Data Store Write3 : DataStoreWrite  DataStoreName=Float_State  IndexOptions=Index vector (dialog)  Indices=1  OutputSizes=1
  Hough Control : Subsystem
  If : If  IfExpression=u1 == 4 | u1 == 5 | u1 == 10 | u1 == 11  ShowElse=off
  MATLAB Function : MATLAB Function  TreatAsAtomicUnit=on
  MATLAB Function1 : MATLAB Function  TreatAsAtomicUnit=on
  Puck State : Constant
  RED+ARM : Subsystem  TreatAsAtomicUnit=on
  RED_Fx : DataStoreWrite  DataStoreName=RED_Fx  IndexOptions=Index vector (dialog)  Indices=1  OutputSizes=1
  RED_Fy : DataStoreWrite  DataStoreName=RED_Fy  IndexOptions=Index vector (dialog)  Indices=1  OutputSizes=1
  RED_Px1 : DataStoreRead  DataStoreName=RED_Px  IndexOptions=Index vector (dialog)  Indices=1  OutputSizes=1
  "RED_Py " : DataStoreRead  DataStoreName=RED_Py  IndexOptions=Index vector (dialog)  Indices=1  OutputSizes=1
  RED_Rz : DataStoreRead  DataStoreName=RED_Rz  IndexOptions=Index vector (dialog)  Indices=1  OutputSizes=1
  RED_Rz Desired : Subsystem
  RED_Tz : DataStoreWrite  DataStoreName=RED_Tz  IndexOptions=Index vector (dialog)  Indices=1  OutputSizes=1
  RED_Tz_RW : DataStoreWrite  DataStoreName=RED_Tz_RW  IndexOptions=Index vector (dialog)  Indices=1  OutputSizes=1
  Subsystem1 : Subsystem
  Subtract : Sum  Inputs=+-
  Subtract2 : Sum  Inputs=+-
  wires:
  Puck State/1 -> Data Store Write3/1
  Hough Control/1(Err) -> Custom Discrete PD (Attitude)/1(ez)
  RED_Rz/1 -> Hough Control/2(Act)
  MATLAB Function1/1(y) -> Subtract2/1
  MATLAB Function/1(x) -> Subtract/1
  Subtract/1 -> Custom Discrete PD (X-Position)/1(ex)
  "RED_Py "/1 -> Subtract2/2
  RED_Rz Desired/1(Ref) -> Hough Control/1(Ref)
  RED_Px1/1 -> Subtract/2
  Subsystem1/1(Out1) -> MATLAB Function/1(t), MATLAB Function1/1(t)
  Subtract2/1 -> Custom Discrete PD (Y-Position)/1(ey)
  Constant4/1 -> RED_Tz_RW/1
  If/1 -> RED+ARM/Action
  Constant1/1 -> If/1
  Custom Discrete PD (Y-Position)/1(Fy) -> RED_Fy/1
  Custom Discrete PD (X-Position)/1(Fx) -> RED_Fx/1
  Custom Discrete PD (Attitude)/1(Tz) -> RED_Tz/1

== system APF_CTL_VIS_Obs_2023a/Phase #3: Experiment/Change RED Behavior/Sub-Phase #4 ==
  note: Additional Blocks
  note: Additional blocks are stored above. Note that to control attitude using the RW, simply replace RED_Tz with RED_Tz_RW.
  note: ARM Control Law - RED
  note: A simple PD control law is used here to command the platform to it's initial position, as defined in the initializer.
  note: PD Control Law - RED
  Action Port : ActionPort  ActionPortLabel=elseif( (u1 < u5 & u1 >= u4))
  BLACK : Subsystem
  BLUE : Subsystem
  CTL : Subsystem
  Constant : Constant  Commented=on  Value=[0;0;0;0;0;0]
  Constant1 : Constant  Value=0
  Constant3 : Constant  Value=platformSelection
  Data Store Write3 : DataStoreWrite  DataStoreName=Float_State  IndexOptions=Index vector (dialog)  Indices=1  OutputSizes=1
  Demux : Demux  Outputs=3
  GDC : Subsystem
  If : If  IfExpression=u1 == 4 | u1 == 5 | u1 == 10 | u1 == 11  ShowElse=off
  Puck State : Constant
  RED : Subsystem
  RED+ARM : Subsystem  TreatAsAtomicUnit=on
  RED_Fx : DataStoreWrite  DataStoreName=RED_Fx  IndexOptions=Index vector (dialog)  Indices=1  OutputSizes=1
  RED_Fy : DataStoreWrite  DataStoreName=RED_Fy  IndexOptions=Index vector (dialog)  Indices=1  OutputSizes=1
  RED_Tz : DataStoreWrite  DataStoreName=RED_Tz  IndexOptions=Index vector (dialog)  Indices=1  OutputSizes=1
  RED_Tz_RW : DataStoreWrite  DataStoreName=RED_Tz_RW  IndexOptions=Index vector (dialog)  Indices=1  OutputSizes=1
  To Workspace2 : ToWorkspace  VariableName=actual_path  SampleTime=-1
  wires:
  Constant1/1 -> RED_Tz_RW/1
  Puck State/1 -> Data Store Write3/1
  If/1 -> RED+ARM/Action
  Constant3/1 -> If/1
  RED/1(state_red) -> GDC/1(state_red), CTL/1(In1), To Workspace2/1
  BLACK/1(state_black) -> GDC/2(state_black)
  BLUE/1(state_blue) -> GDC/4(state_blue)
  BLACK/2(no_IC) -> GDC/3(no_IC)
  GDC/1(Phase) -> CTL/2(Phase)
  GDC/2(Out1) -> CTL/3(In2)
  CTL/1(Control Output) -> Demux/1
  Demux/2 -> RED_Fy/1
  Demux/3 -> RED_Tz/1
  Demux/1 -> RED_Fx/1
  BLUE/2(no_IC) -> GDC/5(Blue?)

== system APF_CTL_VIS_Obs_2023a/Phase #4: Return Home/Change BLACK Behavior/Custom Discrete PD (Attitude) ==
  ez : Inport
  Sum3 : Sum
  kd_tb : Gain  Gain=Kd_tb
  kp_tb : Gain  Gain=Kp_tb
  "x_dot -> x1" : Subsystem
  Tz : Outport  VectorParamsAs1DForOutWhenUnconnected=off
  wires:
  kd_tb/1 -> Sum3/1
  Sum3/1 -> Tz/1
  kp_tb/1 -> Sum3/2
  "x_dot -> x1"/1(dy(t)/dt) -> kd_tb/1
  ez/1 -> "x_dot -> x1"/1(y(t)), kp_tb/1

== system APF_CTL_VIS_Obs_2023a/Phase #4: Return Home/Change BLACK Behavior/Custom Discrete PD (X-Position) ==
  ex : Inport
  Sum3 : Sum
  kd_xb : Gain  Gain=Kd_xb
  kp_xb : Gain  Gain=Kp_xb
  "x_dot -> x1" : Subsystem
  Fx : Outport  VectorParamsAs1DForOutWhenUnconnected=off
  wires:
  kd_xb/1 -> Sum3/1
  ex/1 -> "x_dot -> x1"/1(y(t)), kp_xb/1
  kp_xb/1 -> Sum3/2
  "x_dot -> x1"/1(dy(t)/dt) -> kd_xb/1
  Sum3/1 -> Fx/1

== system APF_CTL_VIS_Obs_2023a/Phase #4: Return Home/Change BLACK Behavior/Custom Discrete PD (Y-Position) ==
  ey : Inport
  Sum3 : Sum
  kd_yb : Gain  Gain=Kd_yb
  kp_yb : Gain  Gain=Kp_yb
  "x_dot -> x1" : Subsystem
  Fy : Outport  VectorParamsAs1DForOutWhenUnconnected=off
  wires:
  kd_yb/1 -> Sum3/1
  Sum3/1 -> Fy/1
  kp_yb/1 -> Sum3/2
  "x_dot -> x1"/1(dy(t)/dt) -> kd_yb/1
  ey/1 -> "x_dot -> x1"/1(y(t)), kp_yb/1

== system APF_CTL_VIS_Obs_2023a/Phase #4: Return Home/Change BLACK Behavior/Hough Control ==
  Ref : Inport
  Act : Inport  Port=2
  MATLAB Function2 : MATLAB Function  TreatAsAtomicUnit=on
  MATLAB Function3 : MATLAB Function  TreatAsAtomicUnit=on
  MATLAB Function4 : MATLAB Function  TreatAsAtomicUnit=on
  Subtract2 : Sum  Inputs=+-
  Err : Outport  VectorParamsAs1DForOutWhenUnconnected=off
  wires:
  MATLAB Function4/1(e_out) -> Err/1
  MATLAB Function2/1(Oy) -> MATLAB Function4/1(Oy)
  Subtract2/1 -> MATLAB Function4/2(e_in)
  MATLAB Function2/2(Ox) -> Subtract2/1
  Act/1 -> MATLAB Function3/1(z)
  Ref/1 -> MATLAB Function2/1(z)
  MATLAB Function3/1(Ox) -> Subtract2/2

== system APF_CTL_VIS_Obs_2023a/Phase #4: Return Home/Change BLUE Behavior/Custom Discrete PD (Attitude) ==
  ez : Inport
  Sum3 : Sum
  kd_tb : Gain  Gain=Kd_tblue
  kp_tb : Gain  Gain=Kp_tblue
  "x_dot -> x1" : Subsystem
  Tz : Outport  VectorParamsAs1DForOutWhenUnconnected=off
  wires:
  kd_tb/1 -> Sum3/1
  Sum3/1 -> Tz/1
  kp_tb/1 -> Sum3/2
  "x_dot -> x1"/1(dy(t)/dt) -> kd_tb/1
  ez/1 -> "x_dot -> x1"/1(y(t)), kp_tb/1

== system APF_CTL_VIS_Obs_2023a/Phase #4: Return Home/Change BLUE Behavior/Custom Discrete PD (X-Position) ==
  ex : Inport
  Sum3 : Sum
  kd_xb : Gain  Gain=Kd_xblue
  kp_xb : Gain  Gain=Kp_xblue
  "x_dot -> x1" : Subsystem
  Fx : Outport  VectorParamsAs1DForOutWhenUnconnected=off
  wires:
  kd_xb/1 -> Sum3/1
  ex/1 -> "x_dot -> x1"/1(y(t)), kp_xb/1
  kp_xb/1 -> Sum3/2
  "x_dot -> x1"/1(dy(t)/dt) -> kd_xb/1
  Sum3/1 -> Fx/1

== system APF_CTL_VIS_Obs_2023a/Phase #4: Return Home/Change BLUE Behavior/Custom Discrete PD (Y-Position) ==
  ey : Inport
  Sum3 : Sum
  kd_yb : Gain  Gain=Kd_yblue
  kp_yb : Gain  Gain=Kp_yblue
  "x_dot -> x1" : Subsystem
  Fy : Outport  VectorParamsAs1DForOutWhenUnconnected=off
  wires:
  kd_yb/1 -> Sum3/1
  Sum3/1 -> Fy/1
  kp_yb/1 -> Sum3/2
  "x_dot -> x1"/1(dy(t)/dt) -> kd_yb/1
  ey/1 -> "x_dot -> x1"/1(y(t)), kp_yb/1

== system APF_CTL_VIS_Obs_2023a/Phase #4: Return Home/Change BLUE Behavior/Hough Control ==
  Ref : Inport
  Act : Inport  Port=2
  MATLAB Function2 : MATLAB Function  TreatAsAtomicUnit=on
  MATLAB Function3 : MATLAB Function  TreatAsAtomicUnit=on
  MATLAB Function4 : MATLAB Function  TreatAsAtomicUnit=on
  Subtract2 : Sum  Inputs=+-
  Err : Outport  VectorParamsAs1DForOutWhenUnconnected=off
  wires:
  MATLAB Function4/1(e_out) -> Err/1
  MATLAB Function2/1(Oy) -> MATLAB Function4/1(Oy)
  Subtract2/1 -> MATLAB Function4/2(e_in)
  MATLAB Function2/2(Ox) -> Subtract2/1
  Act/1 -> MATLAB Function3/1(z)
  Ref/1 -> MATLAB Function2/1(z)
  MATLAB Function3/1(Ox) -> Subtract2/2

== system APF_CTL_VIS_Obs_2023a/Phase #4: Return Home/Change RED Behavior/Custom Discrete PD (Attitude) ==
  ez : Inport
  Sum3 : Sum
  kd_tr : Gain  Gain=Kd_tr
  kp_tr : Gain  Gain=Kp_tr
  "x_dot -> x2" : Subsystem
  Tz : Outport  VectorParamsAs1DForOutWhenUnconnected=off
  wires:
  kd_tr/1 -> Sum3/1
  Sum3/1 -> Tz/1
  kp_tr/1 -> Sum3/2
  "x_dot -> x2"/1(dy(t)/dt) -> kd_tr/1
  ez/1 -> "x_dot -> x2"/1(y(t)), kp_tr/1

== system APF_CTL_VIS_Obs_2023a/Phase #4: Return Home/Change RED Behavior/Custom Discrete PD (X-Position) ==
  ex : Inport
  Sum3 : Sum
  kd_xr : Gain  Gain=Kd_xr
  kp_xr : Gain  Gain=Kp_xr
  "x_dot -> x2" : Subsystem
  Fx : Outport  VectorParamsAs1DForOutWhenUnconnected=off
  wires:
  kd_xr/1 -> Sum3/1
  ex/1 -> "x_dot -> x2"/1(y(t)), kp_xr/1
  kp_xr/1 -> Sum3/2
  "x_dot -> x2"/1(dy(t)/dt) -> kd_xr/1
  Sum3/1 -> Fx/1

== system APF_CTL_VIS_Obs_2023a/Phase #4: Return Home/Change RED Behavior/Custom Discrete PD (Y-Position) ==
  ey : Inport
  Sum3 : Sum
  kd_yr : Gain  Gain=Kd_yr
  kp_yr : Gain  Gain=Kp_yr
  "x_dot -> x2" : Subsystem
  Fy : Outport  VectorParamsAs1DForOutWhenUnconnected=off
  wires:
  kd_yr/1 -> Sum3/1
  Sum3/1 -> Fy/1
  kp_yr/1 -> Sum3/2
  "x_dot -> x2"/1(dy(t)/dt) -> kd_yr/1
  ey/1 -> "x_dot -> x2"/1(y(t)), kp_yr/1

== system APF_CTL_VIS_Obs_2023a/Phase #4: Return Home/Change RED Behavior/Hough Control ==
  Ref : Inport
  Act : Inport  Port=2
  MATLAB Function2 : MATLAB Function  TreatAsAtomicUnit=on
  MATLAB Function3 : MATLAB Function  TreatAsAtomicUnit=on
  MATLAB Function4 : MATLAB Function  TreatAsAtomicUnit=on
  Subtract2 : Sum  Inputs=+-
  Err : Outport  VectorParamsAs1DForOutWhenUnconnected=off
  wires:
  MATLAB Function4/1(e_out) -> Err/1
  MATLAB Function2/1(Oy) -> MATLAB Function4/1(Oy)
  Subtract2/1 -> MATLAB Function4/2(e_in)
  MATLAB Function2/2(Ox) -> Subtract2/1
  Act/1 -> MATLAB Function3/1(z)
  Ref/1 -> MATLAB Function2/1(z)
  MATLAB Function3/1(Ox) -> Subtract2/2
